simulink model "assignment5part2"  (R2022b)
settings: Solver=VariableStepAuto  StartTime=0.0  StopTime=2  MaxStep=1e-3  RelTol=1e-3
settings Model: Creator=aaami  LastModifiedBy=rcmas
settings SolverCC: AlgebraicLoopSolver=TrustRegion
settings DebuggingCC: UnconnectedInputMsg=warning  UnconnectedOutputMsg=warning  UnconnectedLineMsg=warning  SFMachineParentedDataDiag=warning
settings ModelReferenceCC: EnableRefExpFcnMdlSchedulingChecks=on
settings SFSimCC: CustomCodeUndefinedFunction=UseInterfaceOnly

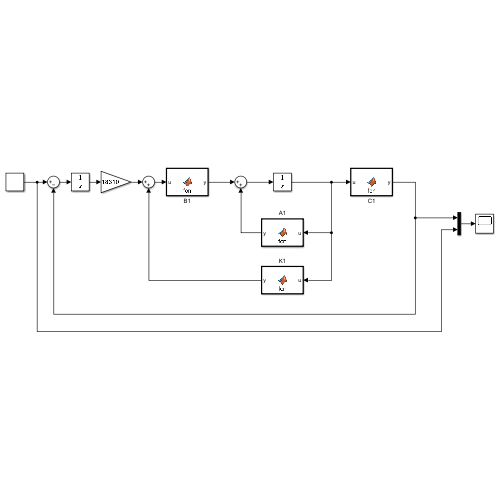
[thumbnail: Simulink's stored preview of the top-level diagram]
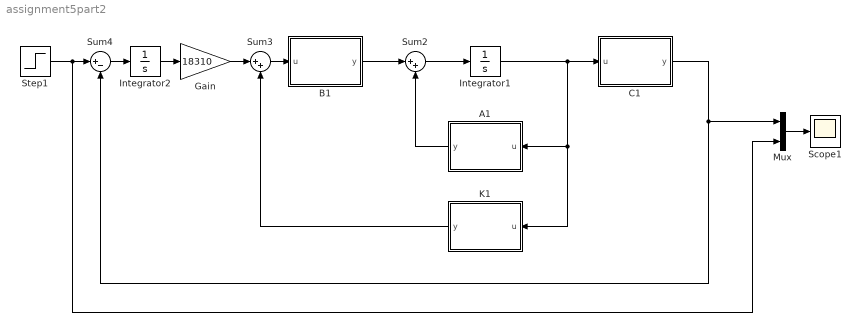
== system assignment5part2 ==
  A1 : MATLAB Function  TreatAsAtomicUnit=on
  B1 : MATLAB Function  TreatAsAtomicUnit=on
  C1 : MATLAB Function  TreatAsAtomicUnit=on
  Gain : Gain  Gain=18310
  Integrator1 : Integrator  InitialCondition=[0;0]
  Integrator2 : Integrator
  K1 : MATLAB Function  TreatAsAtomicUnit=on
  Mux : Mux  Inputs=2
  Scope1 : Scope
  Step1 : Step  Time=0  SampleTime=0
  Sum2 : Sum  Inputs=|++
  Sum3 : Sum  Inputs=|++
  Sum4 : Sum  Inputs=|+-
  wires:
  K1/1(y) -> Sum3/2
  Sum3/1 -> B1/1(u)
  A1/1(y) -> Sum2/2
  B1/1(y) -> Sum2/1
  Sum2/1 -> Integrator1/1
  C1/1(y) -> Mux/1, Sum4/2
  Integrator1/1 -> C1/1(u), A1/1(u), K1/1(u)
  Step1/1 -> Mux/2, Sum4/1
  Gain/1 -> Sum3/1
  Sum4/1 -> Integrator2/1
  Integrator2/1 -> Gain/1
  Mux/1 -> Scope1/1

== matlab function assignment5part2/B1 ==
  data: u input; y output
function y = fcn(u)
B=[0 ; 1];
y = B*u;

== matlab function assignment5part2/C1 ==
  data: u input; y output
function y = fcn(u)
C=[ 1 0];
y = C*u;

== matlab function assignment5part2/K1 ==
  data: u input; y output
function y = fcn(u)
K=-[1780.1 111];
y = K*u;

== matlab function assignment5part2/A1 ==
  data: u input; y output
function y = fcn(u)
A=[0 1
    -3 -5];
y = A*u;
